simulink model "DC_MOTOR_PID"  (R2018a)
settings: Solver=VariableStepAuto  StartTime=0.0  StopTime=80  RelTol=1e-3
model workspace (MAT data in the model file):
  B = 2.21978586253e-20
  J = 0.000193943815709
  K = 0.0137802290227
  L = 0.133562051134
  R = 0.505694900414
libraries: simulink_extras x2, simulink x1
settings Model: Creator=Hazem Elwakeel  LastModifiedBy=abdelrhman

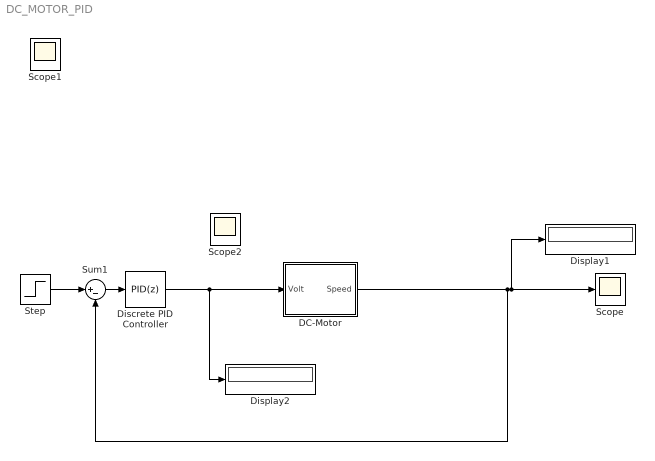
== system DC_MOTOR_PID ==
  "DC-Motor " : Subsystem
  Discrete PID Controller : simulink/Continuous/PID Controller  Controller=PID  TimeDomain=Discrete-time  SampleTime=0.1  IntegratorMethod=Forward Euler  FilterMethod=Forward Euler  Form=Parallel  UseFilter=off  ControllerParametersSource=internal  P=0.000508663294619226  I=0.0101732658923845  D=0.00197146236747095  N=16.1804165352132  InitialConditionSource=internal  InitialConditionForIntegrator=0  InitialConditionForFilter=0  ExternalReset=none  LimitOutput=on  UpperSaturationLimit=12  LowerSaturationLimit=0  LinearizeAsGain=off  AntiWindupMode=none  Kb=1  TrackingMode=off  Kt=1  PParamMin=[]  PParamMax=[]  IParamMin=[]  IParamMax=[]  DParamMin=[]  DParamMax=[]  NParamMin=[]  NParamMax=[]  KbParamMin=[]  KbParamMax=[]  KtParamMin=[]  KtParamMax=[]  POutMin=[]  POutMax=[]  IOutMin=[]  IOutMax=[]  DOutMin=[]  DOutMax=[]  NOutMin=[]  NOutMax=[]  KbOutMin=[]  KbOutMax=[]  KtOutMin=[]  KtOutMax=[]  IntegratorOutMin=[]  IntegratorOutMax=[]  FilterOutMin=[]  FilterOutMax=[]  SumOutMin=[]  SumOutMax=[]  SumI1OutMin=[]  SumI1OutMax=[]  SumI2OutMin=[]  SumI2OutMax=[]  SumI3OutMin=[]  SumI3OutMax=[]  SumDOutMin=[]  SumDOutMax=[]  SaturationOutMin=[]  SaturationOutMax=[]  IntegratorContinuousStateAttributes=''  IntegratorStateMustResolveToSignalObject=off  IntegratorRTWStateStorageClass=Auto  FilterContinuousStateAttributes=''  FilterStateMustResolveToSignalObject=off  FilterRTWStateStorageClass=Auto  DifferentiatorICPrevScaledInput=0  DifferentiatorOutMin=[]  DifferentiatorOutMax=[]  FilterDiffOutCoefMin=[]  FilterDiffOutCoefMax=[]  SumDenOutMin=[]  SumDenOutMax=[]  SumNumOutMin=[]  SumNumOutMax=[]  ReciprocalOutMin=[]  ReciprocalOutMax=[]  DivideOutMin=[]  DivideOutMax=[]  TunerSelectOption=Transfer Function Based (PID Tuner App)
  Display1 : Display
  Display2 : Display
  Scope : Scope
  Scope2 : Scope
  Step : Step  After=500  SampleTime=0.5
  Sum1 : Sum  Inputs=|+-
  Scope1 : Scope
  wires:
  Step/1 -> Sum1/1
  Sum1/1 -> Discrete PID Controller/1
  Discrete PID Controller/1 -> Display2/1, "DC-Motor "/1(Volt)
  "DC-Motor "/1("Speed ") -> Sum1/2, Display1/1, Scope/1

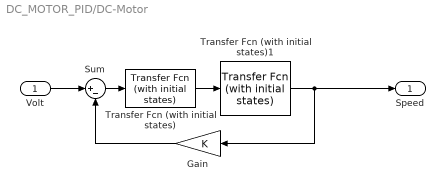
== system DC_MOTOR_PID/DC-Motor  ==
  Volt : Inport
  Gain : Gain  Gain=K
  Sum : Sum  Inputs=|+-
  Transfer Fcn (with initial states) : simulink_extras/Additional Linear/Transfer Fcn (with initial states)  N=[K]  D="[J  B]"  X0=.5
  Transfer Fcn (with initial states)1 : simulink_extras/Additional Linear/Transfer Fcn (with initial states)  N=[1]  D="[L  R]"  X0=.5
  "Speed " : Outport
  wires:
  Transfer Fcn (with initial states)/1 -> Transfer Fcn (with initial states)1/1
  Gain/1 -> Sum/2
  Transfer Fcn (with initial states)1/1 -> "Speed "/1, Gain/1
  Sum/1 -> Transfer Fcn (with initial states)/1
  Volt/1 -> Sum/1
